simulink model "FlFWLvl_VD"  (R2016b)
settings: configuration reference "CodeGenConfigSet" (kept outside this file)
values from neighbouring files (symbols this model uses):
  SigTst_stFlFWLv_C = Calibration.Parameter    [init_FlFWLvl_VD.m]    (also in init_FlFWLvl_VD_SIL.m = Simulink.Parameter)
  SigTst_swtFlFWLv_C = Calibration.Parameter    [init_FlFWLvl_VD.m]    (also in init_FlFWLvl_VD_SIL.m = Simulink.Parameter)
undefined symbols (not defined in the file or in its folder): Switch_conv
settings Model: Creator=胡炎林  LastModifiedBy=胡炎林
settings ConfigSetRef: SourceLocation=Base Workspace

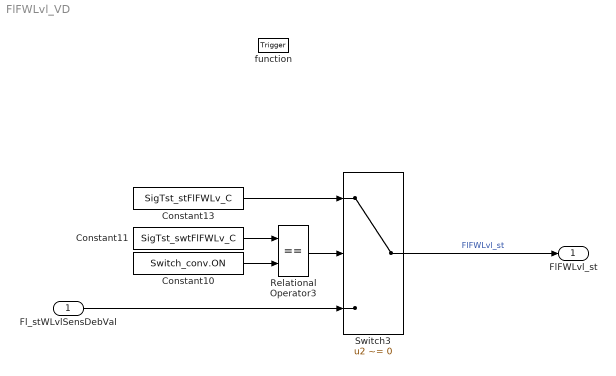
== system FlFWLvl_VD ==
  Fl_stWLvlSensDebVal : Inport  Description=Debounced value of fuel filter water level sensor signal  OutMin=0  OutMax=1  OutDataTypeStr=boolean
  function : TriggerPort  TriggerType=function-call  VariantControl=Variant
  Constant10 : Constant  Value=Switch_conv.ON  OutDataTypeStr=Inherit: Inherit via back propagation
  Constant11 : Constant  Value=SigTst_swtFlFWLv_C  SampleTime=-1
  Constant13 : Constant  Value=SigTst_stFlFWLv_C  OutDataTypeStr=boolean  SampleTime=-1
  Relational Operator3 : RelationalOperator  Operator===  OutDataTypeStr=boolean  RndMeth=Simplest  InputSameDT=on
  Switch3 : Switch  Criteria=u2 ~= 0  InputSameDT=on
  FlFWLvl_st : Outport  Description=status of water in fuel  OutMin=0  OutMax=1  OutDataTypeStr=boolean
  wires:
  Switch3/1 -> FlFWLvl_st/1  "FlFWLvl_st"
  Fl_stWLvlSensDebVal/1 -> Switch3/3
  Constant11/1 -> Relational Operator3/1
  Constant10/1 -> Relational Operator3/2
  Relational Operator3/1 -> Switch3/2
  Constant13/1 -> Switch3/1
